simulink model "simulinkModel"  (R2021b)
settings: Solver=VariableStepAuto  StartTime=0.0  StopTime=10.0  RelTol=1e-3
model workspace (MAT data in the model file):
  LF = 2867.66666667
  LR = 3883.33333333
  RF = 2894
  RR = 3852.33333333
  W = 0.055
  WD = 0.573125555665
  a = 0.306622172281
  b = 0.228377827719
  c = 0.38
  l = 0.535
  m = 13497.3333333
  m_f = 5761.66666667
  m_r = 7735.66666667
  r = 0.0565
settings Model: Creator=Mikeh  LastModifiedBy=Mikeh

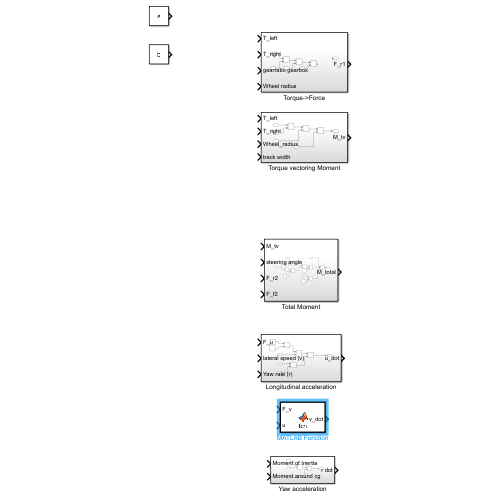
[thumbnail: Simulink's stored preview of the top-level diagram]
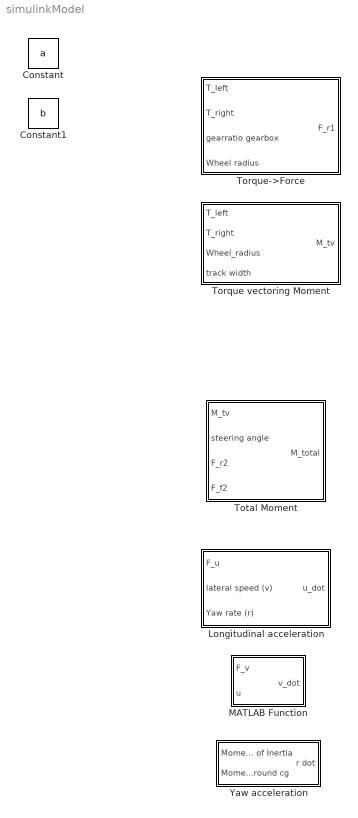
== system simulinkModel ==
  Constant : Constant  Value=a
  Constant1 : Constant  Value=b
  Longitudinal acceleration : Subsystem
  MATLAB Function : MATLAB Function  TreatAsAtomicUnit=on
  Torque vectoring Moment : Subsystem
  Torque->Force : Subsystem
  Total Moment : Subsystem
  Yaw acceleration : Subsystem

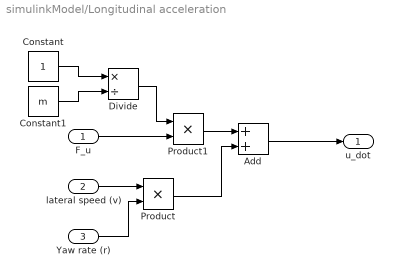
== system simulinkModel/Longitudinal acceleration ==
  F_u : Inport
  lateral speed (v) : Inport  Port=2
  Yaw rate (r) : Inport  Port=3
  Add : Sum
  Constant : Constant
  Constant1 : Constant  Value=m
  Divide : Product  Inputs=*/
  Product : Product
  Product1 : Product
  u_dot : Outport
  wires:
  Constant/1 -> Divide/1
  Constant1/1 -> Divide/2
  lateral speed (v)/1 -> Product/1
  Yaw rate (r)/1 -> Product/2
  F_u/1 -> Product1/2
  Divide/1 -> Product1/1
  Product1/1 -> Add/1
  Product/1 -> Add/2
  Add/1 -> u_dot/1

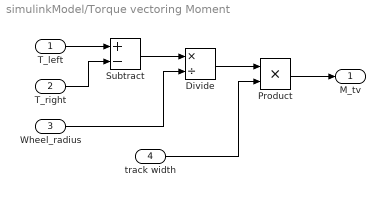
== system simulinkModel/Torque vectoring Moment ==
  T_left : Inport
  T_right : Inport  Port=2
  Wheel_radius : Inport  Port=3
  track width : Inport  Port=4
  Divide : Product  Inputs=*/
  Product : Product
  Subtract : Sum  Inputs=+-
  M_tv : Outport
  wires:
  T_left/1 -> Subtract/1
  T_right/1 -> Subtract/2
  Subtract/1 -> Divide/1
  Wheel_radius/1 -> Divide/2
  Divide/1 -> Product/1
  track width/1 -> Product/2
  Product/1 -> M_tv/1

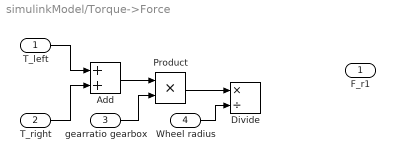
== system simulinkModel/Torque->Force ==
  T_left : Inport
  T_right : Inport  Port=2
  gearratio gearbox : Inport  Port=3
  Wheel radius : Inport  Port=4
  Add : Sum
  Divide : Product  Inputs=*/
  Product : Product
  F_r1 : Outport
  wires:
  T_left/1 -> Add/1
  T_right/1 -> Add/2
  Add/1 -> Product/1
  gearratio gearbox/1 -> Product/2
  Product/1 -> Divide/1
  Wheel radius/1 -> Divide/2

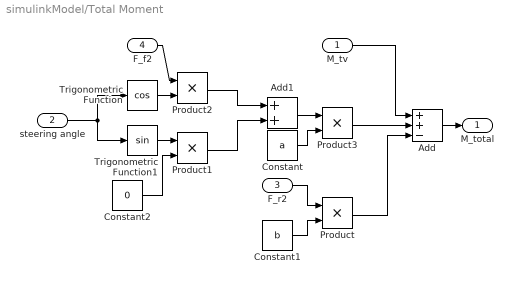
== system simulinkModel/Total Moment ==
  M_tv : Inport
  steering angle : Inport  Port=2
  F_r2 : Inport  Port=3
  F_f2 : Inport  Port=4
  Add : Sum  Inputs=++-
  Add1 : Sum
  Constant : Constant  Value=a
  Constant1 : Constant  Value=b
  Constant2 : Constant  Value=0
  Product{,1..3} (4 alike) : Product
  Trigonometric Function : Trigonometry  Operator=cos
  Trigonometric Function1 : Trigonometry
  M_total : Outport
  wires:
  Constant1/1 -> Product/2
  F_r2/1 -> Product/1
  Add/1 -> M_total/1
  Product/1 -> Add/3
  M_tv/1 -> Add/1
  steering angle/1 -> Trigonometric Function1/1, Trigonometric Function/1
  Trigonometric Function1/1 -> Product1/1
  Constant2/1 -> Product1/2
  Trigonometric Function/1 -> Product2/2
  F_f2/1 -> Product2/1
  Product2/1 -> Add1/1
  Product1/1 -> Add1/2
  Add1/1 -> Product3/1
  Product3/1 -> Add/2
  Constant/1 -> Product3/2

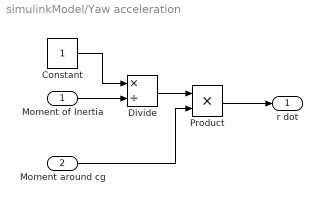
== system simulinkModel/Yaw acceleration ==
  Moment of Inertia : Inport
  Moment around cg : Inport  Port=2
  Constant : Constant
  Divide : Product  Inputs=*/
  Product : Product
  r dot : Outport
  wires:
  Moment of Inertia/1 -> Divide/2
  Constant/1 -> Divide/1
  Divide/1 -> Product/1
  Moment around cg/1 -> Product/2
  Product/1 -> r dot/1

== matlab function simulinkModel/MATLAB Function ==
  data: F_v input; u input; v_dot output
function v_dot = fcn(F_v, u)
v_dot = (1/m)*F_v - u *r;
